simulink model "GFM_L_Filter"  (R2016a)
settings: Solver=ode1  SolverMode=SingleTasking  StartTime=0.0  StopTime=5  FixedStep=Time_Step2  MaxStep=1e-5  RelTol=1e-3
PreLoadFcn:
  | GFM_L_Filter_Init;
InitFcn:
  | GFM_L_Filter_Init;
undefined symbols (not defined in the file): GRD00_Lg, GRD00_Rg, Time_Step2
libraries: powerlib x7, GFM_Lib x2, Source_Lib x1
settings Model: Creator=Frederic_Colas  LastModifiedBy=Frederic_Colas
settings DebuggingCC: UnconnectedInputMsg=none  UnconnectedOutputMsg=none  UnconnectedLineMsg=none  SFUnexpectedBacktrackingDiag=error  SFNoUnconditionalDefaultTransitionDiag=error
settings HardwareCC: ProdWordSize=32  ProdHWDeviceType=Specified
settings GRTTargetCC: TargetLangStandard=C99 (ISO)
settings ConfigComp: CovMetricSettings=dwe  CovSaveCumulativeToWorkspaceVar=off  CovSaveSingleToWorkspaceVar=off  CovExternalEMLEnable=on
settings SimscapeCC: SimscapeNormalizeSystem=off

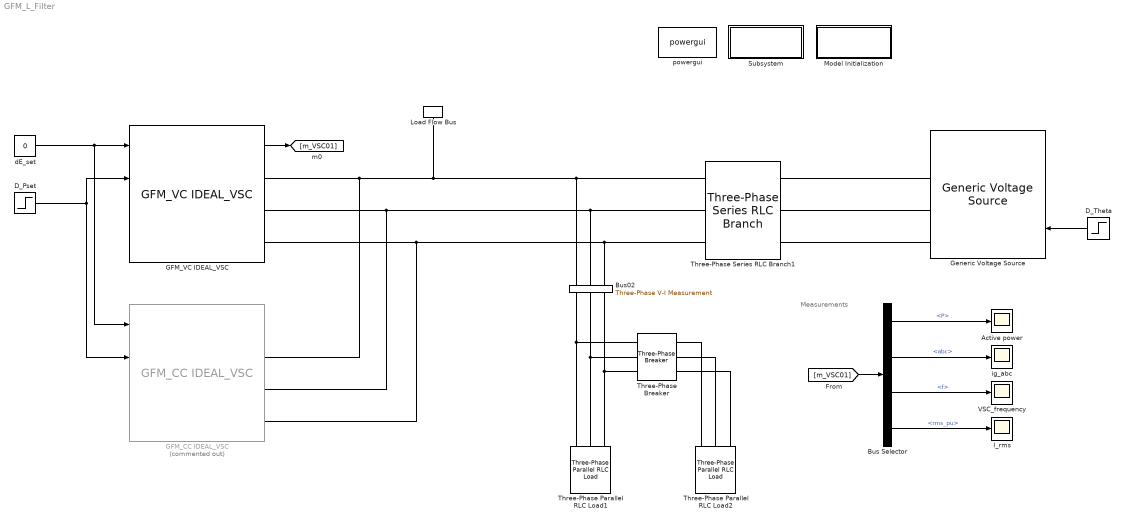
== system GFM_L_Filter ==
  note: Measurements
  Active power : Scope
  Bus Selector : BusSelector  OutputSignals=P,Ig.abc,f,Ig.rms_pu
  "Bus02 " : powerlib/Measurements/Three-Phase V-I Measurement  VoltageMeasurement=no  SetLabelV=off  LabelV=Vabc  Vpu=off  VpuLL=off  CurrentMeasurement=no  SetLabelI=off  LabelI=Iabc  Ipu=off  Pbase=100e6  Vbase=500e3  OutputType=Complex  PhasorSimulation=off  PSBequivalent=0
  D_Pset : Step  After=0.4  SampleTime=0
  D_Theta : Step  Time=4  After=0.05  SampleTime=0
  GFM_CC IDEAL_VSC : GFM_Lib/GFM_CC IDEAL_VSC  Commented=on  fn=50  Sn=1000e6  Pn=1000e6  Udcn=640e3  Output_Delay=375e-6  Un1=320e3  Un2=400e3  Rt_pu=0.005  Lt_pu=0.15  Lm_pu=10000  Rm_pu=10000  DC_Link=Perfect DC Source  H_DC=inf  H_DC_sav=inf  wn_PLL=500  zeta_PLL=1  Val_Freq_Support=off  R_percent=4  dLc_pu=0  Rv=0.09  W_TVR=60  I_max_pu=1.2  Tr_I_max=10  Tau_fCC=0.01  wn_CC=1000  Kffi=on  Filtre_FF=on  w_ff=1000  Advanced=on  gainpopup=With Inertia  wn_Inertia_Less=5/(2*pi)  Param_Inertia=VSM  H_GFo=5  zeta_GFo=1  LFpopup=PQ  P0=0.3  Q0=0  V0=1.005  Theta0=5.6773
  GFM_VC IDEAL_VSC : GFM_Lib/GFM_VC IDEAL_VSC  fn=50  Sn=1000e6  Pn=1000e6  Udcn=640e3  Output_Delay=375e-6  Un1=320e3  Un2=400e3  Rt_pu=0.005  Lt_pu=0.15  Lm_pu=500  Rm_pu=500  DC_Link=Perfect DC Source  H_DC=inf  H_DC_sav=40  wn_PLL=50  zeta_PLL=1  Val_Freq_Support=off  R_percent=4  dLc_pu=0  Rv=0.09  W_TVR=60  I_max_pu=1.2  wn_I_max=300  I_Max_TVI_pu=1.2  DX_DR=5  Advanced=on  gainpopup=With Inertia  wn_Inertia_Less=10  Param_Inertia=VSM  H_GFo=5  zeta_GFo=1  LFpopup=PQ  P0=0.3  Q0=0  V0=1.005  Theta0=5.6773
  Generic Voltage Source : Source_Lib/Generic Voltage Source  SourceNature_str=INFINITE  fn=50  Sn=1e9  Un=Ug  H_s=5  DroopOnOff=on  R_percent=4  TN=1  TD=2  Time_Step=Time_Step  LFpopup=Swing  P0=-0.19688  Q0=0.019573  V0=1  Theta0=0
  I_rms : Scope
  Load Flow Bus : powerlib/Measurements/Load Flow Bus  LConnTagsString=a  Phases=single  Connectors=on one side  ID=BUS_1  Vbase=400e3  Vref=1  Vangle=0  VLF=1.005  VLFb=1  VLFc=1  angleLF=5.677  angleLFb=0  angleLFc=0
  Model Initialization : Subsystem  mask(Model Functions){InitFcnX=GFM_L_Filter_Init;, prel=on, posl=off, inif=on, strf=off}
      mask prompts: InitFcnX "Initialisation"; prel "Preload Function"; posl "PostLoad Function"; inif "InitFcn"; strf "StartFcn"
      mask init:
      | currentBlock = gcb;
      | root = bdroot(currentBlock);
      | 
      | if ~strcmp(get_param(root,'BlockDiagramType'),'library')
      |     if prel==1
      |         set_param(root, 'PreLoadFcn', InitFcnX);
      |     else
      |         set_param(root, 'PreLoadFcn', '');
      |     end
      |     if inif==1
      |         set_param(root, 'InitFcn', InitFcnX);
      |     else
      |         set_param(root, 'InitFcn', '');
      |     end
      |     if strf==1
      |         set_param(root, 'StartFcn', InitFcnX);
      |     else
      |         set_param(root, 'StartFcn', '');
      |     end
      |     if posl==1
      |         set_param(root, 'PostLoadFcn', InitFcnX);
      |     else
      |         set_param(root, 'PostLoadFcn', '');
      |     end
      | end
      | 
      | pos = get_param(currentBlock, 'Position');
      | width = pos(3) - pos(1); height = pos(4) - pos(2);
      | txt = [ upper(root) '\n' '- InitFcn. . . . . '  get_param(root, 'InitFcn') ];
      settings: CopyFcn=set_param(gcb,'LinkStatus','none')
      mask Display:
      | %text(5, height*0.5, txt, 'horizontalAlignment', 'left', 'verticalAlignment', 'middle') ;
      | color('blue'),disp('Initialization Function\nParameters')
  Subsystem : Subsystem
      settings: OpenFcn=LoadFlow_VSC
      mask Display: color('blue'),disp('Update Loadflow')
  Three-Phase Parallel RLC Load1 : powerlib/Elements/Three-Phase Parallel RLC Load  LConnTagsString=A|B|C  Configuration=Y (grounded)  NominalVoltage=Ug  Vabc=[1e3 1e3 1e3]  Vabcp=[1e3 1e3 1e3]  NominalFrequency=fb  UnbalancedPower=off  ActivePower=100e6  InductivePower=0  CapacitivePower=0  Pabc=[10e3 9e3 11e3]  QLabc=[100 90 110]  QCabc=[100 90 110]  Pabcp=[10e3 9e3 11e3]  QLabcp=[100 90 110]  QCabcp=[100 90 110]  Measurements=None  LoadType=constant Z
  Three-Phase Parallel RLC Load2 : powerlib/Elements/Three-Phase Parallel RLC Load  LConnTagsString=A|B|C  Configuration=Y (grounded)  NominalVoltage=Ug  Vabc=[1e3 1e3 1e3]  Vabcp=[1e3 1e3 1e3]  NominalFrequency=fb  UnbalancedPower=off  ActivePower=1000e6  InductivePower=0  CapacitivePower=0  Pabc=[10e3 9e3 11e3]  QLabc=[100 90 110]  QCabc=[100 90 110]  Pabcp=[10e3 9e3 11e3]  QLabcp=[100 90 110]  QCabcp=[100 90 110]  Measurements=None  LoadType=constant Z
  Three-Phase Series RLC Branch1 : powerlib/Elements/Three-Phase Series RLC Branch  LConnTagsString=A|B|C  RConnTagsString=A|B|C  BranchType=RL  Resistance=GRD00_Rg  Inductance=GRD00_Lg  Capacitance=1e-6  Measurements=None
  Three-Phase Breaker : powerlib/Elements/Three-Phase Breaker  InitialState=open  SwitchA=on  SwitchB=on  SwitchC=on  SwitchTimes=3  External=off  BreakerResistance=0.01  SnubberResistance=1e6  SnubberCapacitance=inf  Measurements=None
  VSC_frequency : Scope
  dE_set : Constant  Value=0
  ig_abc : Scope
  powergui : powerlib/powergui  Priority=1  SimulationMode=Discrete  SampleTime=Time_Step2  frequency=60  Iterations=50  frequencyindice=50  Pbase=1000000000  ErrMax=1e-6  UnitsV=kV  UnitsW=MW  buscounter=0  FunctionMessages=off  echomessages=off  EnableUseOfTLC=off  CurrentSourceSwitches=off  DisableSnubberDevices=off  DisableRonSwitches=off  DisableVfSwitches=off  DisplayEquations=off  AutomaticDiscreteSolvers=off  SolverType=Tustin/Backward Euler (TBE)  Interpol=off  ExternalGateDelay=off  methode=off  Ts=100  x0status=blocks  SPID=on  SwTol=0  HookPort=off  NonlinearTolerance=1e-4  nMaxIteration=100  ContinueOnMaxIteration=off  RestoreLinks=warning  ResistiveCurrentMeasurement=off  Frange=[0:2:500]  Ylog=off  Xlog=on  ShowGrid=off  save=off  variable=ZData  structure=0  ZoomFFT=off  StartTime=0.0  cycles=1  DisplayStyle=1  fundamental=60  FreqAxis=off  MaxFrequency=1000  frequencyindicesteady=1  RmsSteady=1  display=off
  wires:
  [m_VSC01] -> Bus Selector/1
  Bus Selector/1 -> Active power/1  "<P>"
  Bus Selector/4 -> I_rms/1  "<rms_pu>"
  Bus Selector/2 -> ig_abc/1  "<abc>"
  Bus Selector/3 -> VSC_frequency/1  "<f>"
  dE_set/1 -> GFM_CC IDEAL_VSC/1, GFM_VC IDEAL_VSC/1
  D_Pset/1 -> GFM_VC IDEAL_VSC/2, GFM_CC IDEAL_VSC/2
  GFM_VC IDEAL_VSC/1 -> [m_VSC01]
  D_Theta/1 -> Generic Voltage Source/2
  connections:
  "Bus02 "/LConn3 -- Load Flow Bus/LConn1 -- GFM_CC IDEAL_VSC/RConn1 -- GFM_VC IDEAL_VSC/RConn1 -- Three-Phase Series RLC Branch1/LConn1
  "Bus02 "/LConn1 -- GFM_CC IDEAL_VSC/RConn3 -- GFM_VC IDEAL_VSC/RConn3 -- Three-Phase Series RLC Branch1/LConn3
  "Bus02 "/LConn2 -- GFM_CC IDEAL_VSC/RConn2 -- GFM_VC IDEAL_VSC/RConn2 -- Three-Phase Series RLC Branch1/LConn2
  Generic Voltage Source/RConn1 -- Three-Phase Series RLC Branch1/RConn1
  Generic Voltage Source/RConn2 -- Three-Phase Series RLC Branch1/RConn2
  Generic Voltage Source/RConn3 -- Three-Phase Series RLC Branch1/RConn3
  Three-Phase Parallel RLC Load1/LConn2 -- "Bus02 "/RConn2 -- Three-Phase Breaker/LConn2
  Three-Phase Parallel RLC Load1/LConn3 -- "Bus02 "/RConn1 -- Three-Phase Breaker/LConn3
  Three-Phase Parallel RLC Load1/LConn1 -- "Bus02 "/RConn3 -- Three-Phase Breaker/LConn1
  Three-Phase Parallel RLC Load2/LConn3 -- Three-Phase Breaker/RConn3
  Three-Phase Parallel RLC Load2/LConn2 -- Three-Phase Breaker/RConn2
  Three-Phase Breaker/RConn1 -- Three-Phase Parallel RLC Load2/LConn1

== system GFM_L_Filter/Model Initialization ==

== system GFM_L_Filter/Subsystem ==
